simulink model "SignalExample"  (R2016b)
settings: Solver=FixedStepAuto  StartTime=0.0  StopTime=100  FixedStep=1  RelTol=1e-3
settings Model: Creator=gauti  LastModifiedBy=gauti

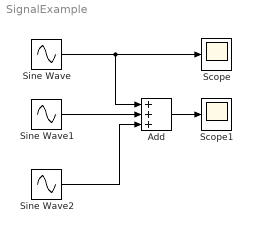
== system SignalExample ==
  Add : Sum  Inputs=+++
  Scope : Scope
  Scope1 : Scope
  Sine Wave : Sin  SampleTime=0
  Sine Wave1 : Sin  Frequency=0.8  SampleTime=0
  Sine Wave2 : Sin  Frequency=1.2  SampleTime=0
  wires:
  Sine Wave/1 -> Add/1, Scope/1
  Sine Wave1/1 -> Add/2
  Sine Wave2/1 -> Add/3
  Add/1 -> Scope1/1
